simulink model "PI_Controller_Discrete"  (R2023a)
settings: Solver=VariableStepAuto  StartTime=0.0  StopTime=10.0  RelTol=1e-3
undefined symbols (not defined in the file or in its folder): a, b, K, r, Tsamp
settings Model: Creator=m260477  LastModifiedBy=m260477

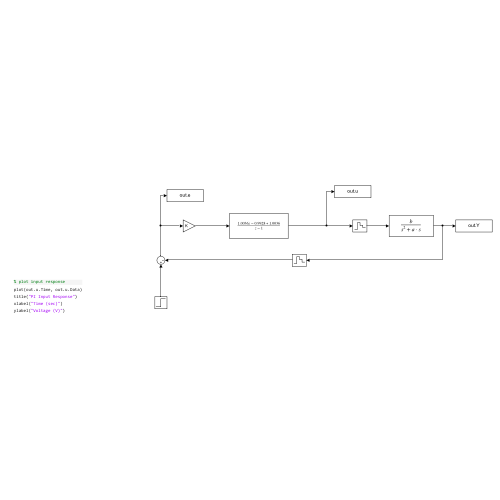
[thumbnail: Simulink's stored preview of the top-level diagram]
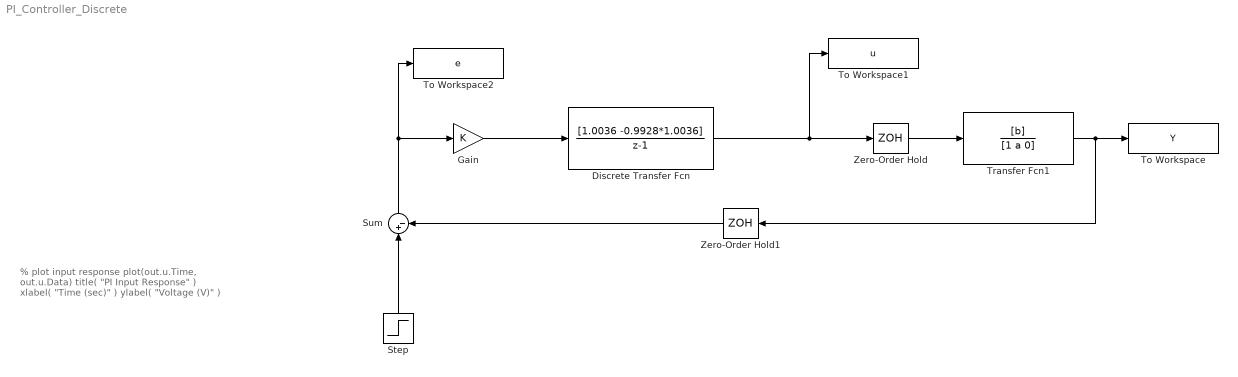
== system PI_Controller_Discrete ==
  note: % plot input response
      | plot(out.u.Time, out.u.Data)
      | title( "PI Input Response" )
      | xlabel( "Time (sec)" )
      | ylabel( "Voltage (V)" )
  Discrete Transfer Fcn : DiscreteTransferFcn  Numerator=[1.0036 -0.9928*1.0036]  Denominator=[1 -1]  SampleTime=Tsamp
  Gain : Gain  Gain=K
  Step : Step  Time=0  After=r  SampleTime=0
  Sum : Sum  Inputs=|+-
  To Workspace : ToWorkspace  VariableName=Y  SaveFormat=Timeseries  SampleTime=-1
  To Workspace1 : ToWorkspace  VariableName=u  SaveFormat=Timeseries  SampleTime=-1
  To Workspace2 : ToWorkspace  VariableName=e  SaveFormat=Timeseries  SampleTime=-1
  Transfer Fcn1 : TransferFcn  Numerator=[b]  Denominator=[1 a 0]
  Zero-Order Hold : ZeroOrderHold  SampleTime=Tsamp
  Zero-Order Hold1 : ZeroOrderHold  SampleTime=Tsamp
  wires:
  Gain/1 -> Discrete Transfer Fcn/1
  Sum/1 -> To Workspace2/1, Gain/1
  Discrete Transfer Fcn/1 -> To Workspace1/1, Zero-Order Hold/1
  Transfer Fcn1/1 -> Zero-Order Hold1/1, To Workspace/1
  Step/1 -> Sum/1
  Zero-Order Hold/1 -> Transfer Fcn1/1
  Zero-Order Hold1/1 -> Sum/2
